simulink model "SeparatelyExcited_DC_Motor_Sim"  (R2022b)
settings: Solver=ode23tb  StartTime=0.0  StopTime=inf  MaxStep=.001  RelTol=1e-3
values from neighbouring files (symbols this model uses):
  B = .01    (= 0.01)    [SeparatelyExcited_DC_Motor_Parameter.m]
  J = 5    [SeparatelyExcited_DC_Motor_Parameter.m]
  Kphi = 1.6    [SeparatelyExcited_DC_Motor_Parameter.m]
  La = .1    (= 0.1)    [SeparatelyExcited_DC_Motor_Parameter.m]
  Ra = .5    (= 0.5)    [SeparatelyExcited_DC_Motor_Parameter.m]
  TL = 20    [SeparatelyExcited_DC_Motor_Parameter.m]
  Va = 200    [SeparatelyExcited_DC_Motor_Parameter.m]
settings Model: Creator=MOHAMED  LastModifiedBy=MOHAMED

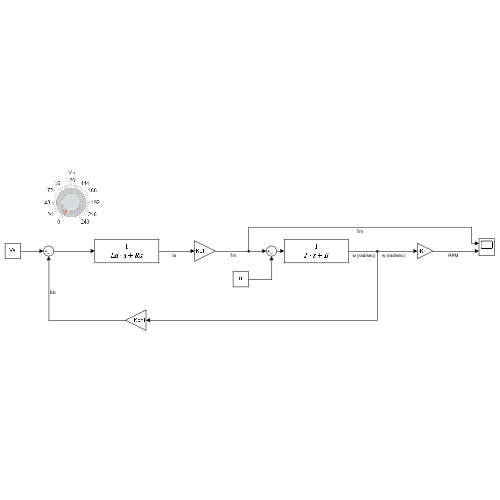
[thumbnail: Simulink's stored preview of the top-level diagram]
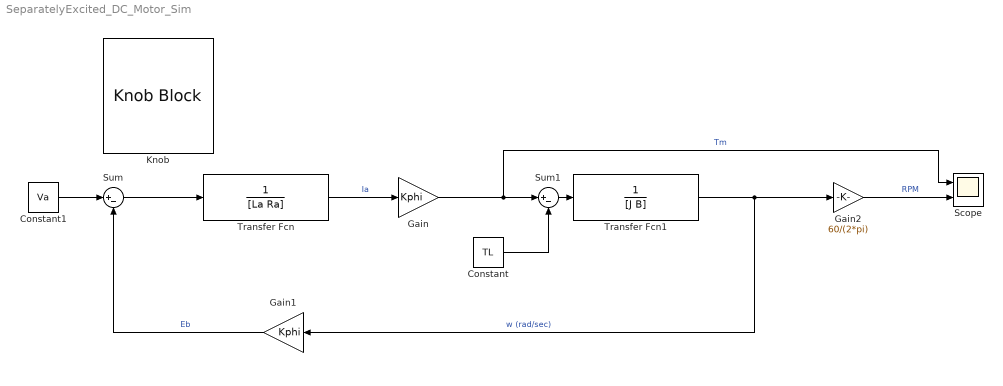
== system SeparatelyExcited_DC_Motor_Sim ==
  Constant : Constant  Value=TL
  Constant1 : Constant  Value=Va
  Gain : Gain  Gain=Kphi
  Gain1 : Gain  Gain=Kphi
  Gain2 : Gain  Gain=60/(2*pi)
  Knob : KnobBlock  ScaleMax=240
  Scope : Scope  NumInputPorts=2
  Sum : Sum  Inputs=|+-
  Sum1 : Sum  Inputs=|+-
  Transfer Fcn : TransferFcn  Denominator=[La Ra]
  Transfer Fcn1 : TransferFcn  Denominator=[J B]
  wires:
  Gain1/1 -> Sum/2  "Eb"
  Sum/1 -> Transfer Fcn/1
  Transfer Fcn/1 -> Gain/1  "Ia"
  Gain/1 -> Scope/1, Sum1/1  "Tm"
  Sum1/1 -> Transfer Fcn1/1
  Transfer Fcn1/1 -> Gain1/1, Gain2/1  "w (rad/sec)"
  Gain2/1 -> Scope/2  "RPM"
  Constant/1 -> Sum1/2
  Constant1/1 -> Sum/1
